simulink model "nominal_tracking"  (R2020b)
settings: Solver=ode45  StartTime=0.0  StopTime=5  RelTol=1e-3
undefined symbols (not defined in the file or in its folder): A0, B0, C0, D0, daq, degs2rpm, denHwa, denHws, drv, GAMMA, gbox, H0, J0, mld, mot, N_u, N_x, numHwa, numHws, PHI, rads2rpm, sens, step_size, T, tau_hat
settings Model: Creator=utente  LastModifiedBy=utente
settings DataIOCC: ReturnWorkspaceOutputs=off

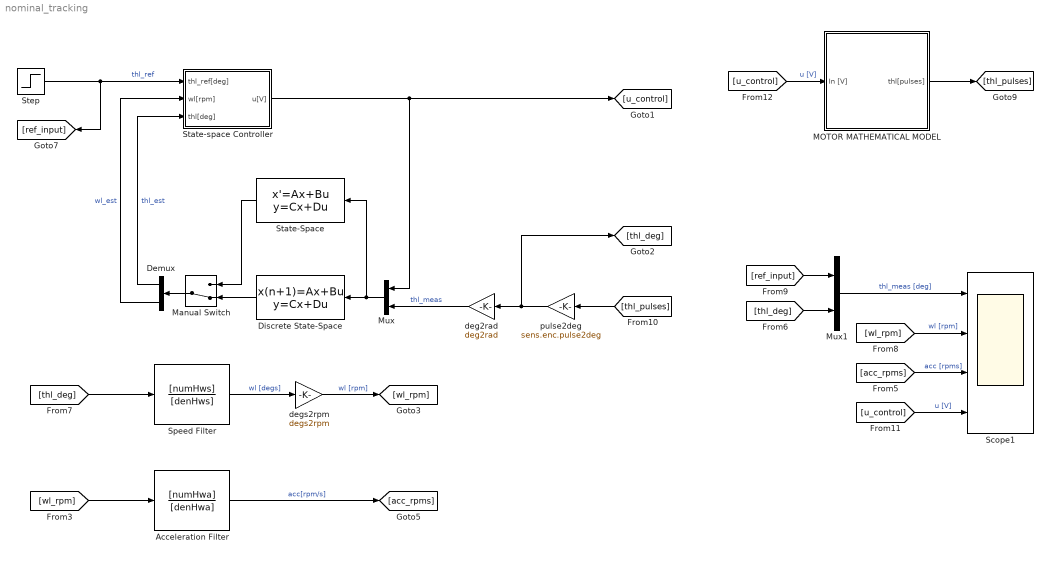
== system nominal_tracking ==
  Acceleration Filter : TransferFcn  Numerator=[numHwa]  Denominator=[denHwa]
  Demux : Demux  Outputs=2
  Discrete State-Space : DiscreteStateSpace  A=PHI  B=GAMMA  C=H0  D=J0  SampleTime=T
  MOTOR MATHEMATICAL MODEL : Subsystem
  Manual Switch : ManualSwitch  CurrentSetting=0
  Mux : Mux  Inputs=2
  Mux1 : Mux  Inputs=2
  Scope1 : Scope  NumInputPorts=4
  Speed Filter : TransferFcn  Numerator=[numHws]  Denominator=[denHws]
  State-Space : StateSpace  A=A0  B=B0  C=C0  D=D0  InitialCondition=0
  State-space Controller : Subsystem
  Step : Step  After=step_size  SampleTime=0
  deg2rad : Gain  Gain=deg2rad
  degs2rpm : Gain  Gain=degs2rpm
  pulse2deg : Gain  Gain=sens.enc.pulse2deg
  wires:
  State-space Controller/1(u[V]) -> [u_control], Mux/1
  [thl_pulses] -> pulse2deg/1
  Step/1 -> [ref_input], State-space Controller/1(thl_ref[deg])  "thl_ref"
  pulse2deg/1 -> [thl_deg], deg2rad/1
  deg2rad/1 -> Mux/2  "thl_meas"
  Demux/1 -> State-space Controller/3(thl[deg])  "thl_est"
  Demux/2 -> State-space Controller/2(wl[rpm])  "wl_est"
  Mux/1 -> Discrete State-Space/1, State-Space/1
  Manual Switch/1 -> Demux/1
  Discrete State-Space/1 -> Manual Switch/2
  State-Space/1 -> Manual Switch/1
  degs2rpm/1 -> [wl_rpm]  "wl [rpm]"
  [ref_input] -> Mux1/1
  Speed Filter/1 -> degs2rpm/1  "wl [degs]"
  [thl_deg] -> Mux1/2
  Acceleration Filter/1 -> [acc_rpms]  "acc[rpm/s]"
  [thl_deg] -> Speed Filter/1
  [acc_rpms] -> Scope1/3  "acc [rpms]"
  [wl_rpm] -> Scope1/2  "wl [rpm]"
  Mux1/1 -> Scope1/1  "thl_meas [deg]"
  [u_control] -> Scope1/4  "u [V]"
  [wl_rpm] -> Acceleration Filter/1
  MOTOR MATHEMATICAL MODEL/1(thl[pulses]) -> [thl_pulses]
  [u_control] -> MOTOR MATHEMATICAL MODEL/1(In [V])  "u [V]"

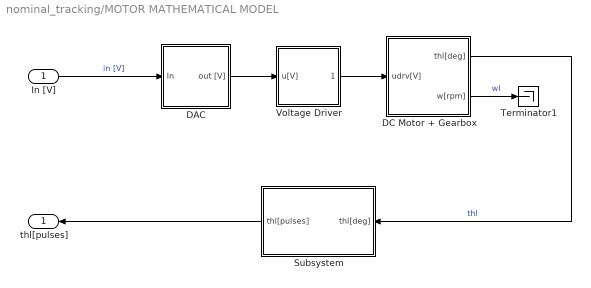
== system nominal_tracking/MOTOR MATHEMATICAL MODEL ==
  In [V] : Inport
  DAC : Subsystem
  DC Motor + Gearbox : Subsystem
  Subsystem : Subsystem
  Terminator1 : Terminator
  Voltage Driver : Subsystem
  thl[pulses] : Outport
  wires:
  In [V]/1 -> DAC/1(In)  "in [V]"
  DC Motor + Gearbox/1(thl[deg]) -> Subsystem/1(thl[deg])  "thl"
  DAC/1(out [V]) -> Voltage Driver/1(u[V])
  DC Motor + Gearbox/2(w[rpm]) -> Terminator1/1  "wl"
  Subsystem/1(thl[pulses]) -> thl[pulses]/1
  Voltage Driver/1(udrv[V]) -> DC Motor + Gearbox/1(udrv[V])

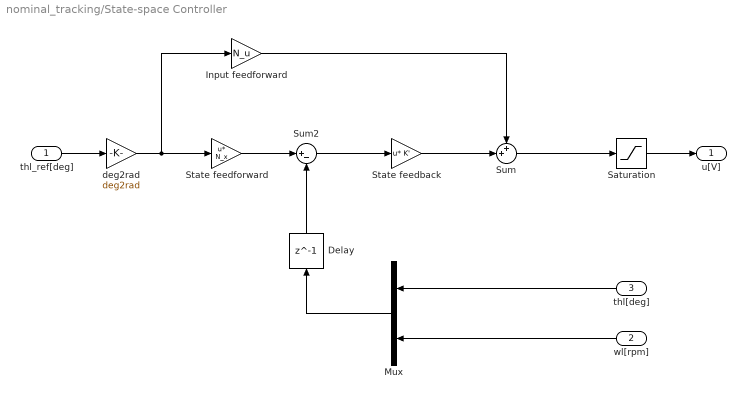
== system nominal_tracking/State-space Controller ==
  thl_ref[deg] : Inport
  wl[rpm] : Inport  Port=2
  thl[deg] : Inport  Port=3
  Delay : Delay  DelayLength=1  InitialCondition=0
  Input feedforward : Gain  Gain=N_u
  Mux : Mux  Inputs=2
  Saturation : Saturate  UpperLimit=10  LowerLimit=-10
  State feedback : Gain  Gain=K'  Multiplication=Matrix(u*K)
  "State feedforward\t" : Gain  Gain=N_x  Multiplication=Matrix(u*K)
  Sum : Sum  Inputs=++|
  Sum2 : Sum  Inputs=|+-
  deg2rad : Gain  Gain=deg2rad
  u[V] : Outport
  wires:
  thl_ref[deg]/1 -> deg2rad/1
  deg2rad/1 -> Input feedforward/1, "State feedforward\t"/1
  State feedback/1 -> Sum/2
  "State feedforward\t"/1 -> Sum2/1
  Sum2/1 -> State feedback/1
  Input feedforward/1 -> Sum/1
  Sum/1 -> Saturation/1
  Saturation/1 -> u[V]/1
  thl[deg]/1 -> Mux/1
  wl[rpm]/1 -> Mux/2
  Mux/1 -> Delay/1
  Delay/1 -> Sum2/2

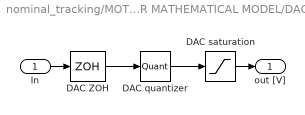
== system nominal_tracking/MOTOR MATHEMATICAL MODEL/DAC ==
  In : Inport
  DAC quantizer : Quantizer  QuantizationInterval=daq.dac.q
  DAC saturation : Saturate  UpperLimit=daq.dac.fs  LowerLimit=-daq.dac.fs
  DAC ZOH : ZeroOrderHold  SampleTime=0.001
  out [V] : Outport
  wires:
  DAC saturation/1 -> out [V]/1
  In/1 -> DAC ZOH/1
  DAC quantizer/1 -> DAC saturation/1
  DAC ZOH/1 -> DAC quantizer/1

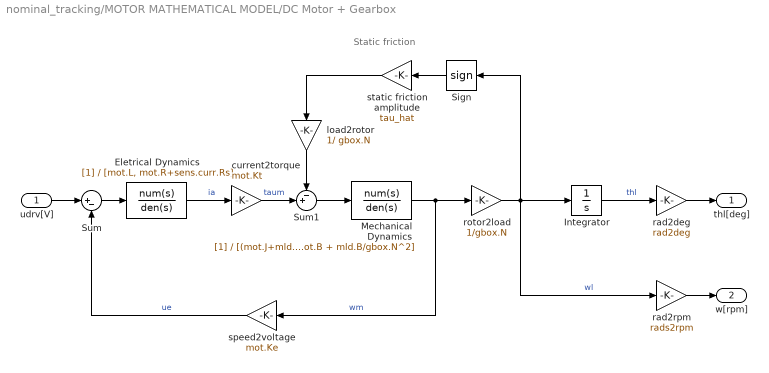
== system nominal_tracking/MOTOR MATHEMATICAL MODEL/DC Motor + Gearbox ==
  note: Static friction
  udrv[V] : Inport
  Eletrical Dynamics : TransferFcn  Denominator=[mot.L, mot.R+sens.curr.Rs]
  Integrator : Integrator
  Mechanical Dynamics : TransferFcn  Denominator=[(mot.J+mld.J/gbox.N^2), mot.B + mld.B/gbox.N^2]
  Sign : Signum  ZeroCross=off
  Sum : Sum  Inputs=|+-
  Sum1 : Sum  Inputs=-+|
  current2torque : Gain  Gain=mot.Kt
  load2rotor : Gain  Gain=1/ gbox.N
  rad2deg : Gain  Gain=rad2deg
  "rad2rpm " : Gain  Gain=rads2rpm
  rotor2load : Gain  Gain=1/gbox.N
  speed2voltage : Gain  Gain=mot.Ke
  static friction amplitude : Gain  Gain=tau_hat
  thl[deg] : Outport  VectorParamsAs1DForOutWhenUnconnected=off
  w[rpm] : Outport  Port=2  VectorParamsAs1DForOutWhenUnconnected=off
  wires:
  Eletrical Dynamics/1 -> current2torque/1  "ia"
  udrv[V]/1 -> Sum/1
  Sum/1 -> Eletrical Dynamics/1
  current2torque/1 -> Sum1/2  "taum"
  Sum1/1 -> Mechanical Dynamics/1
  Mechanical Dynamics/1 -> rotor2load/1, speed2voltage/1  "wm"
  rotor2load/1 -> Integrator/1, "rad2rpm "/1, Sign/1  "wl"
  Integrator/1 -> rad2deg/1  "thl"
  rad2deg/1 -> thl[deg]/1
  "rad2rpm "/1 -> w[rpm]/1
  Sign/1 -> static friction amplitude/1
  speed2voltage/1 -> Sum/2  "ue"
  static friction amplitude/1 -> load2rotor/1
  load2rotor/1 -> Sum1/1

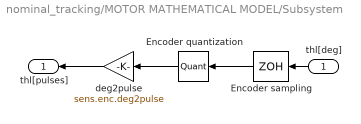
== system nominal_tracking/MOTOR MATHEMATICAL MODEL/Subsystem ==
  thl[deg] : Inport
  Encoder quantization : Quantizer  QuantizationInterval=sens.enc.pulse2deg
  Encoder sampling : ZeroOrderHold  SampleTime=-1
  deg2pulse : Gain  Gain=sens.enc.deg2pulse
  thl[pulses] : Outport
  wires:
  thl[deg]/1 -> Encoder sampling/1
  Encoder quantization/1 -> deg2pulse/1
  Encoder sampling/1 -> Encoder quantization/1
  deg2pulse/1 -> thl[pulses]/1

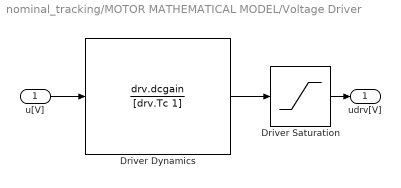
== system nominal_tracking/MOTOR MATHEMATICAL MODEL/Voltage Driver ==
  u[V] : Inport
  Driver Dynamics : TransferFcn  Numerator=drv.dcgain  Denominator=[drv.Tc 1]
  Driver Saturation : Saturate  UpperLimit=12  LowerLimit=-12
  udrv[V] : Outport
  wires:
  u[V]/1 -> Driver Dynamics/1
  Driver Saturation/1 -> udrv[V]/1
  Driver Dynamics/1 -> Driver Saturation/1
